simulink library "lib_energy_storage"  (Simulink 4.00)
undefined symbols (not defined in the file): air_cp, amb_tmp, cyc_mph, enable_stop, ess_cap_scale, ess_cb, ess_cc, ess_coulombic_eff, ess_init_soc, ess_max_ah_cap, ess_max_p, ess_max_p_soc, ess_max_soc, ess_max_volts, ess_min_soc, ess_min_volts, ess_MMi, ess_MMo, ess_mod_airflow, ess_mod_cp, ess_mod_cpm, ess_mod_init_tmp, ess_module_mass, ess_module_num, ess_on, ess_parallel_mod_num, ess_res_scale_coef, ess_res_scale_fun, ess_set_tmp, ess_soc, ess_th_calc, ess_th_res, ess_th_res_off, ess_th_res_on, ess_tmp, ess_voc, fund_byu, fund_byuop, mc_min_volts, saber_air_temp, Saber_Battery_IO_File, saber_init_soc, saber_init_temp, saber_init_voc, saber_k_cb, saber_k_cc, saber_k_rc, saber_k_re, saber_k_rt, saber_k_soc, t_soc, time_step
libraries: simulink3 x16, lib_energy_storage x3
(part 2 of 3)

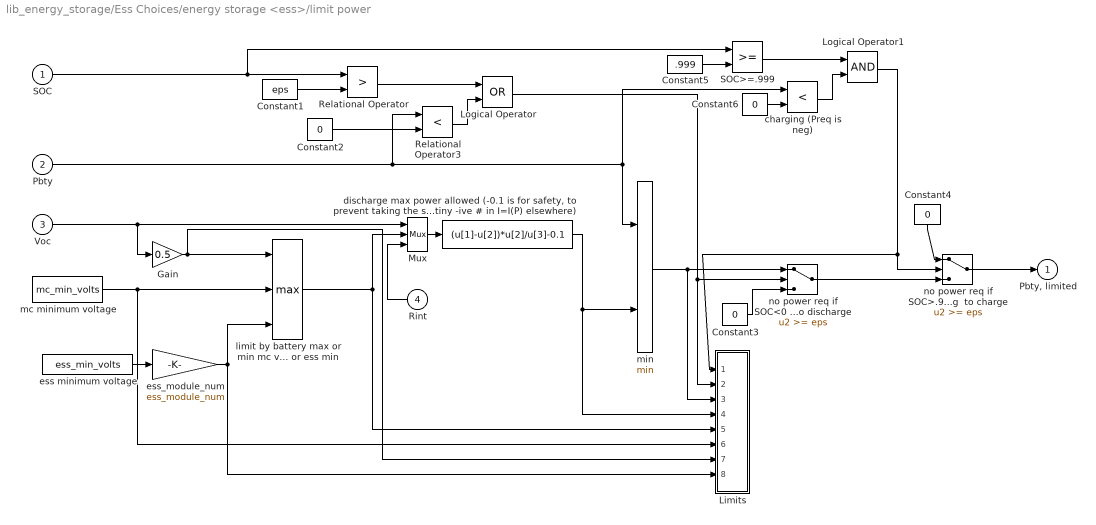
== system lib_energy_storage/Ess Choices/energy storage <ess>/limit power ==
  SOC : Inport  Port=1  LatchInput=off
  Pbty : Inport  Port=2  LatchInput=off
  Voc : Inport  Port=3  LatchInput=off
  Rint : Inport  Orientation=left  Port=4  LatchInput=off
  Constant1 : Constant  Value=eps
  Constant2 : Constant  Value=0
  Constant3 : Constant  Value=0
  Constant4 : Constant  Orientation=down  Value=0
  Constant5 : Constant  Value=.999
  Constant6 : Constant  Value=0
  Gain : Gain  Gain=0.5  Multiplication=Element-wise(K.*u)  SaturateOnIntegerOverflow=on
  Limits : Subsystem
      settings: RTWFcnNameOpts=Auto  RTWFileNameOpts=Auto
  Logical Operator : Logic  Operator=OR  Inputs=2
  Logical Operator1 : Logic  Operator=AND  Inputs=2
  Mux : Mux  Inputs=3
      settings: DisplayOption=none
  Relational Operator : RelationalOperator  Operator=>
  Relational Operator3 : RelationalOperator  Operator=<
  SOC>=.999 : RelationalOperator  Operator=>=
  charging (Preq is neg) : RelationalOperator  Operator=<
  "discharge max power allowed (-0.1 is for safety, to prevent taking the square of a tiny -ive # in I=I(P) elsewhere)" : Fcn  Expr=(u[1]-u[2])*u[2]/u[3]-0.1
  ess minimum voltage : Constant  Value=ess_min_volts
  ess_module_num : Gain  Gain=ess_module_num  Multiplication=Element-wise(K.*u)  SaturateOnIntegerOverflow=on
  limit by battery max or min mc voltage or ess min : MinMax  Function=max  Inputs=3
  mc minimum voltage : Constant  Value=mc_min_volts
  min : MinMax  Function=min  Inputs=2
  no power req if SOC<0 and trying  to discharge : Switch  Threshold=eps
  no power req if SOC>.999 and trying  to charge : Switch  Threshold=eps
  "Pbty, limited" : Outport  Port=1  InitialOutput=0
  wires:
  Logical Operator1/1 -> Limits/1(SOC  high limited), no power req if SOC>.999 and trying  to charge/2
  no power req if SOC>.999 and trying  to charge/1 -> "Pbty, limited"/1
  no power req if SOC<0 and trying  to discharge/1 -> no power req if SOC>.999 and trying  to charge/3
  Constant4/1 -> no power req if SOC>.999 and trying  to charge/1
  Constant5/1 -> SOC>=.999/2
  charging (Preq is neg)/1 -> Logical Operator1/2
  Constant6/1 -> charging (Preq is neg)/2
  SOC>=.999/1 -> Logical Operator1/1
  SOC/1 -> SOC>=.999/1, Relational Operator/1
  ess_module_num/1 -> Limits/8(V ess_min_volts), limit by battery max or min mc voltage or ess min/3
  ess minimum voltage/1 -> ess_module_num/1
  Gain/1 -> Limits/7(V battery (.5Voc)), limit by battery max or min mc voltage or ess min/1
  Rint/1 -> Mux/3
  mc minimum voltage/1 -> Limits/6(V mc_min_volts), limit by battery max or min mc voltage or ess min/2
  "discharge max power allowed (-0.1 is for safety, to prevent taking the square of a tiny -ive # in I=I(P) elsewhere)"/1 -> min/2, Limits/4(power bat limited)
  limit by battery max or min mc voltage or ess min/1 -> Limits/5(V used), Mux/2
  Mux/1 -> "discharge max power allowed (-0.1 is for safety, to prevent taking the square of a tiny -ive # in I=I(P) elsewhere)"/1
  min/1 -> Limits/3(power req), no power req if SOC<0 and trying  to discharge/1
  Voc/1 -> Gain/1, Mux/1
  Logical Operator/1 -> Limits/2(not SOC  low limited), no power req if SOC<0 and trying  to discharge/2
  Constant3/1 -> no power req if SOC<0 and trying  to discharge/3
  Relational Operator3/1 -> Logical Operator/2
  Constant2/1 -> Relational Operator3/2
  Pbty/1 -> charging (Preq is neg)/1, min/1, Relational Operator3/1
  Relational Operator/1 -> Logical Operator/1
  Constant1/1 -> Relational Operator/2

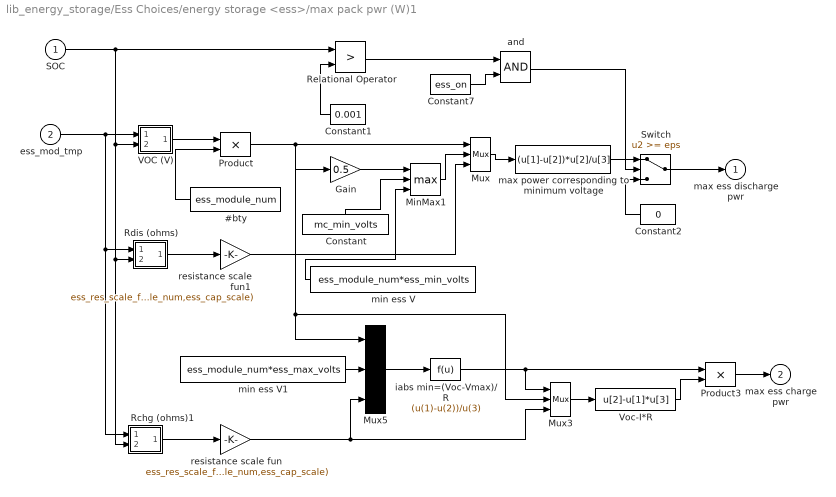
== system lib_energy_storage/Ess Choices/energy storage <ess>/max pack pwr (W)1 ==
  SOC : Inport  Port=1  LatchInput=off
  ess_mod_tmp : Inport  Port=2  LatchInput=off
  #bty : Constant  Orientation=left  Value=ess_module_num
  Constant : Constant  Orientation=up  Value=mc_min_volts
  Constant1 : Constant  Orientation=left  Value=0.001
  Constant2 : Constant  Orientation=left  Value=0
  Constant7 : Constant  Value=ess_on
  Gain : Gain  Gain=0.5  Multiplication=Element-wise(K.*u)  SaturateOnIntegerOverflow=on
  MinMax1 : MinMax  Function=max  Inputs=3
  Mux : Mux  Inputs=3
      settings: DisplayOption=none
  Mux3 : Mux  Inputs=3
      settings: DisplayOption=none
  Mux5 : Mux  Inputs=3
      settings: DisplayOption=none
  Product : Product  Inputs=2  Multiplication=Element-wise(.*)  SaturateOnIntegerOverflow=on
  Product3 : Product  Inputs=2  Multiplication=Element-wise(.*)  SaturateOnIntegerOverflow=on
  Rchg (ohms)1 : Subsystem  mask(2-D Table Lookup){@1=ess_tmp, @2=ess_soc, @3=ess_r_chg}
      mask prompts: @1 "X Index"; @2 "Y Index"; @3 "Table"
      mask help:
      | Two Dimensional Table Lookup
      | The first input corresponds to X Index and the second input corresponds to the Y Index
      mask init:
      | xindex=@1; yindex=@2; table=@3; sftab2chk(xindex,yindex,table);
      settings: RTWFcnNameOpts=Auto  RTWFileNameOpts=Auto
      mask Help: This block returns a linearly interpolated intersection from the table using the X index (which corresponds to the rows of the table) and the Y index (which corresponds to the columns of the table).  Extrapolation is used.
      mask Display: plot(-10,-10,110,110,[90,50,10],[90,40,30],[90,50,10],[50,26,20],[90,50,10],[22,13,10])
  Rdis (ohms) : Subsystem  mask(2-D Table Lookup){@1=ess_tmp, @2=ess_soc, @3=ess_r_dis}
      mask prompts: @1 "X Index"; @2 "Y Index"; @3 "Table"
      mask help:
      | Two Dimensional Table Lookup
      | The first input corresponds to X Index and the second input corresponds to the Y Index
      mask init:
      | xindex=@1; yindex=@2; table=@3; sftab2chk(xindex,yindex,table);
      settings: RTWFcnNameOpts=Auto  RTWFileNameOpts=Auto
      mask Help: This block returns a linearly interpolated intersection from the table using the X index (which corresponds to the rows of the table) and the Y index (which corresponds to the columns of the table).  Extrapolation is used.
      mask Display: plot(-10,-10,110,110,[90,50,10],[90,40,30],[90,50,10],[50,26,20],[90,50,10],[22,13,10])
  Relational Operator : RelationalOperator  Operator=>
  Switch : Switch  Threshold=eps
  VOC (V) : Subsystem  mask(2-D Table Lookup){@1=ess_tmp, @2=ess_soc, @3=ess_voc}
      mask prompts: @1 "X Index"; @2 "Y Index"; @3 "Table"
      mask help:
      | Two Dimensional Table Lookup
      | The first input corresponds to X Index and the second input corresponds to the Y Index
      mask init:
      | xindex=@1; yindex=@2; table=@3; sftab2chk(xindex,yindex,table);
      settings: RTWFcnNameOpts=Auto  RTWFileNameOpts=Auto
      mask Help: This block returns a linearly interpolated intersection from the table using the X index (which corresponds to the rows of the table) and the Y index (which corresponds to the columns of the table).  Extrapolation is used.
      mask Display: plot(-10,-10,110,110,[90,50,10],[90,40,30],[90,50,10],[50,26,20],[90,50,10],[22,13,10])
  Voc-I*R : Fcn  Expr=u[2]-u[1]*u[3]
  and : Logic  Operator=AND  Inputs=2
  iabs min=(Voc-Vmax)/R : Fcn  Expr=(u(1)-u(2))/u(3)
  max power corresponding to minimum voltage : Fcn  Expr=(u[1]-u[2])*u[2]/u[3]
  min ess V : Constant  Orientation=left  Value=ess_module_num*ess_min_volts
  min ess V1 : Constant  Value=ess_module_num*ess_max_volts
  resistance scale fun : Gain  Gain=ess_res_scale_fun(ess_res_scale_coef,ess_module_num,ess_cap_scale)  Multiplication=Element-wise(K.*u)  SaturateOnIntegerOverflow=on
  resistance scale fun1 : Gain  Gain=ess_res_scale_fun(ess_res_scale_coef,ess_module_num,ess_cap_scale)  Multiplication=Element-wise(K.*u)  SaturateOnIntegerOverflow=on
  max ess discharge pwr : Outport  Port=1  InitialOutput=0
  max ess charge pwr : Outport  Port=2  InitialOutput=0
  wires:
  Constant7/1 -> and/2
  Relational Operator/1 -> and/1
  and/1 -> Switch/2
  min ess V/1 -> MinMax1/3
  ess_mod_tmp/1 -> VOC (V)/1(x0), Rdis (ohms)/1(x0), Rchg (ohms)1/1(x0)
  Constant1/1 -> Relational Operator/2
  Constant/1 -> MinMax1/2
  Mux/1 -> max power corresponding to minimum voltage/1
  Gain/1 -> MinMax1/1
  MinMax1/1 -> Mux/2
  Product/1 -> Mux/1, Gain/1, Mux5/1, Mux3/2
  resistance scale fun1/1 -> Mux/3
  VOC (V)/1(table out) -> Product/1
  Rdis (ohms)/1(table out) -> resistance scale fun1/1
  max power corresponding to minimum voltage/1 -> Switch/1
  Constant2/1 -> Switch/3
  SOC/1 -> Relational Operator/1, VOC (V)/2(y0), Rdis (ohms)/2(y0), Rchg (ohms)1/2(y0)
  Switch/1 -> max ess discharge pwr/1
  min ess V1/1 -> Mux5/2
  Mux5/1 -> iabs min=(Voc-Vmax)/R/1
  Mux3/1 -> Voc-I*R/1
  iabs min=(Voc-Vmax)/R/1 -> Mux3/1, Product3/1
  Voc-I*R/1 -> Product3/2
  Product3/1 -> max ess charge pwr/1
  resistance scale fun/1 -> Mux5/3, Mux3/3
  Rchg (ohms)1/1(table out) -> resistance scale fun/1
  #bty/1 -> Product/2

== system lib_energy_storage/Ess Choices/energy storage <ess>/pack Voc, Rint ==
  SOC (prev) : Inport  Port=1  LatchInput=off
  req'd battery power (W) : Inport  Port=2  LatchInput=off
  mod tmp   (C) : Inport  Port=3  LatchInput=off
  #bty : Constant  Value=ess_module_num
  Product : Product  Inputs=2  Multiplication=Element-wise(.*)  SaturateOnIntegerOverflow=on
  Rchg (ohms) : Subsystem  mask(2-D Table Lookup){@1=ess_tmp, @2=ess_soc, @3=ess_r_chg}
      mask prompts: @1 "X Index"; @2 "Y Index"; @3 "Table"
      mask help:
      | Two Dimensional Table Lookup
      | The first input corresponds to X Index and the second input corresponds to the Y Index
      mask init:
      | xindex=@1; yindex=@2; table=@3; sftab2chk(xindex,yindex,table);
      settings: RTWFcnNameOpts=Auto  RTWFileNameOpts=Auto
      mask Help: This block returns a linearly interpolated intersection from the table using the X index (which corresponds to the rows of the table) and the Y index (which corresponds to the columns of the table).  Extrapolation is used.
      mask Display: plot(-10,-10,110,110,[90,50,10],[90,40,30],[90,50,10],[50,26,20],[90,50,10],[22,13,10])
  Rdis (ohms) : Subsystem  mask(2-D Table Lookup){@1=ess_tmp, @2=ess_soc, @3=ess_r_dis}
      mask prompts: @1 "X Index"; @2 "Y Index"; @3 "Table"
      mask help:
      | Two Dimensional Table Lookup
      | The first input corresponds to X Index and the second input corresponds to the Y Index
      mask init:
      | xindex=@1; yindex=@2; table=@3; sftab2chk(xindex,yindex,table);
      settings: RTWFcnNameOpts=Auto  RTWFileNameOpts=Auto
      mask Help: This block returns a linearly interpolated intersection from the table using the X index (which corresponds to the rows of the table) and the Y index (which corresponds to the columns of the table).  Extrapolation is used.
      mask Display: plot(-10,-10,110,110,[90,50,10],[90,40,30],[90,50,10],[50,26,20],[90,50,10],[22,13,10])
  Switch : Switch  Threshold=0
  VOC (V) : Subsystem  mask(2-D Table Lookup){@1=ess_tmp, @2=ess_soc, @3=ess_voc}
      mask prompts: @1 "X Index"; @2 "Y Index"; @3 "Table"
      mask help:
      | Two Dimensional Table Lookup
      | The first input corresponds to X Index and the second input corresponds to the Y Index
      mask init:
      | xindex=@1; yindex=@2; table=@3; sftab2chk(xindex,yindex,table);
      settings: RTWFcnNameOpts=Auto  RTWFileNameOpts=Auto
      mask Help: This block returns a linearly interpolated intersection from the table using the X index (which corresponds to the rows of the table) and the Y index (which corresponds to the columns of the table).  Extrapolation is used.
      mask Display: plot(-10,-10,110,110,[90,50,10],[90,40,30],[90,50,10],[50,26,20],[90,50,10],[22,13,10])
  resistance scale fun : Gain  Gain=ess_res_scale_fun(ess_res_scale_coef,ess_module_num,ess_cap_scale)  Multiplication=Element-wise(K.*u)  SaturateOnIntegerOverflow=on
  resistance scale fun1 : Gain  Gain=ess_res_scale_fun(ess_res_scale_coef,ess_module_num,ess_cap_scale)  Multiplication=Element-wise(K.*u)  SaturateOnIntegerOverflow=on
  pack open- circuit voltage : Outport  Port=1  InitialOutput=0
  pack resistance : Outport  Port=2  InitialOutput=0
  wires:
  mod tmp   (C)/1 -> Rchg (ohms)/1(x0), Rdis (ohms)/1(x0), VOC (V)/1(x0)
  SOC (prev)/1 -> Rchg (ohms)/2(y0), Rdis (ohms)/2(y0), VOC (V)/2(y0)
  req'd battery power (W)/1 -> Switch/2
  VOC (V)/1(table out) -> Product/1
  Product/1 -> pack open- circuit voltage/1
  #bty/1 -> Product/2
  Switch/1 -> pack resistance/1
  Rdis (ohms)/1(table out) -> resistance scale fun/1
  resistance scale fun/1 -> Switch/1
  Rchg (ohms)/1(table out) -> resistance scale fun1/1
  resistance scale fun1/1 -> Switch/3

== system lib_energy_storage/Ess Choices/energy storage <ess>/stop sim ==
  SOC : Inport  Port=1  LatchInput=off
  Enable : EnablePort
  Const : Constant  Orientation=up  Value=.001
  Relational Operator : RelationalOperator  Operator=<
  Stop Simulation : Stop
  wires:
  Relational Operator/1 -> Stop Simulation/1
  SOC/1 -> Relational Operator/1
  Const/1 -> Relational Operator/2

== system lib_energy_storage/Ess Choices/energy storage <ess> RC/Allow simulation to stop based on  low SOC ==
  SOC : Inport  Port=1  LatchInput=off
  Enable : EnablePort
  Const : Constant  Orientation=up  Value=.001
  Relational Operator : RelationalOperator  Operator=<
  Stop Simulation : Stop
  wires:
  Relational Operator/1 -> Stop Simulation/1
  SOC/1 -> Relational Operator/1
  Const/1 -> Relational Operator/2

== system lib_energy_storage/Ess Choices/energy storage <ess> RC/Block NOTES ==
  note: This block models the energy storage system as an SOC-dependent voltage
      | in series with an SOC- and current direction-dependent internal resistance.
      | SOC is computed assuming that A-h capacity is constant, but limited
      | such that a minimum voltage is never exceeded (replacing the
      | previous Peukert relationship which underpredicted battery capacity).
      |
      | Discharge power is limited here so as not to bring the bus (battery pack) voltage below
      | the minimum controller voltage or the minimum battery voltage and so as to allow
      | the solution of the quadratic eq'n for discharge current.
      |
      | Charge current is limited to ensure the voltage does not exceed a maximum
      | voltage
      |
      | Positive current is discharge current in the convention used here.
      | Power loss is computed as I*R+losses due to Coulombic (in)efficiency.
      |
      | Thermal modeling of the battery performance is modeled in the
      | OCV, Rint, and capacity.

== system lib_energy_storage/Ess Choices/energy storage <ess> RC/Model Parameters ==
  SOC : Inport  Port=1  LatchInput=off
  Ess Temp : Inport  Port=2  LatchInput=off
  Preq : Inport  Port=3  LatchInput=off
  Terminator : Terminator
  cb : Lookup  InputValues=ess_tmp  OutputValues=ess_cb
  cc : Lookup  InputValues=ess_tmp  OutputValues=ess_cc
  rc : Subsystem  mask(2-D Table Lookup){@1=ess_tmp, @2=ess_soc, @3=ess_rc}
      mask prompts: @1 "X Index"; @2 "Y Index"; @3 "Table"
      mask help:
      | Two Dimensional Table Lookup
      | The first input corresponds to X Index and the second input corresponds to the Y Index
      mask init:
      | xindex=@1; yindex=@2; table=@3; sftab2chk(xindex,yindex,table);
      settings: RTWFcnNameOpts=Auto  RTWFileNameOpts=Auto
      mask Help: This block returns a linearly interpolated intersection from the table using the X index (which corresponds to the rows of the table) and the Y index (which corresponds to the columns of the table).  Extrapolation is used.
      mask Display: plot(-10,-10,110,110,[90,50,10],[90,40,30],[90,50,10],[50,26,20],[90,50,10],[22,13,10])
  re : Subsystem  mask(2-D Table Lookup){@1=ess_tmp, @2=ess_soc, @3=ess_re}
      mask prompts: @1 "X Index"; @2 "Y Index"; @3 "Table"
      mask help:
      | Two Dimensional Table Lookup
      | The first input corresponds to X Index and the second input corresponds to the Y Index
      mask init:
      | xindex=@1; yindex=@2; table=@3; sftab2chk(xindex,yindex,table);
      settings: RTWFcnNameOpts=Auto  RTWFileNameOpts=Auto
      mask Help: This block returns a linearly interpolated intersection from the table using the X index (which corresponds to the rows of the table) and the Y index (which corresponds to the columns of the table).  Extrapolation is used.
      mask Display: plot(-10,-10,110,110,[90,50,10],[90,40,30],[90,50,10],[50,26,20],[90,50,10],[22,13,10])
  rt : Subsystem  mask(2-D Table Lookup){@1=ess_tmp, @2=ess_soc, @3=ess_rt}
      mask prompts: @1 "X Index"; @2 "Y Index"; @3 "Table"
      mask help:
      | Two Dimensional Table Lookup
      | The first input corresponds to X Index and the second input corresponds to the Y Index
      mask init:
      | xindex=@1; yindex=@2; table=@3; sftab2chk(xindex,yindex,table);
      settings: RTWFcnNameOpts=Auto  RTWFileNameOpts=Auto
      mask Help: This block returns a linearly interpolated intersection from the table using the X index (which corresponds to the rows of the table) and the Y index (which corresponds to the columns of the table).  Extrapolation is used.
      mask Display: plot(-10,-10,110,110,[90,50,10],[90,40,30],[90,50,10],[50,26,20],[90,50,10],[22,13,10])
  Cb : Outport  Port=1  InitialOutput=0
  Cc : Outport  Port=2  InitialOutput=0
  Re : Outport  Port=3  InitialOutput=0
  Rc : Outport  Port=4  InitialOutput=0
  Rt : Outport  Port=5  InitialOutput=0
  wires:
  rc/1(table out) -> Rc/1
  rt/1(table out) -> Rt/1
  re/1(table out) -> Re/1
  cc/1 -> Cc/1
  cb/1 -> Cb/1
  SOC/1 -> rt/2(y0), rc/2(y0), re/2(y0)
  Preq/1 -> Terminator/1
  Ess Temp/1 -> rt/1(x0), rc/1(x0), re/1(x0), cc/1, cb/1

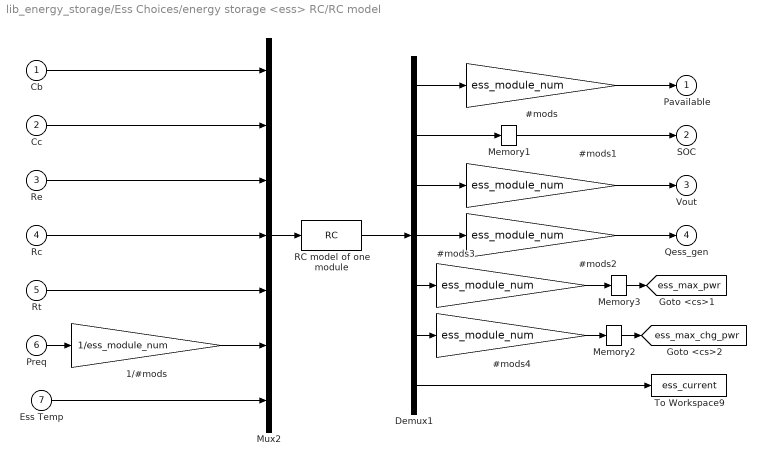
== system lib_energy_storage/Ess Choices/energy storage <ess> RC/RC model ==
  Cb : Inport  Port=1  LatchInput=off
  Cc : Inport  Port=2  LatchInput=off
  Re : Inport  Port=3  LatchInput=off
  Rc : Inport  Port=4  LatchInput=off
  Rt : Inport  Port=5  LatchInput=off
  Preq : Inport  Port=6  LatchInput=off
  Ess Temp : Inport  Port=7  LatchInput=off
  #mods{,1..4} (5 alike) : Gain  Gain=ess_module_num  Multiplication=Element-wise(K.*u)  SaturateOnIntegerOverflow=on
  1/#mods : Gain  Gain=1/ess_module_num  Multiplication=Element-wise(K.*u)  SaturateOnIntegerOverflow=on
  Demux1 : Demux  Outputs=7  BusSelectionMode=off
  Memory1 : Memory  X0=ess_init_soc  InheritSampleTime=off
      settings: RTWStateStorageClass=Auto
  Memory2 : Memory  X0=0  InheritSampleTime=off
      settings: RTWStateStorageClass=Auto
  Memory3 : Memory  X0=0  InheritSampleTime=off
      settings: RTWStateStorageClass=Auto
  Mux2 : Mux  Inputs=7
      settings: DisplayOption=none
  RC model of one module : S-Function  FunctionName=RC  Parameters=ess_min_volts,ess_max_volts,mc_min_volts/ess_module_num,ess_soc,ess_tmp,ess_voc,ess_init_soc,ess_mod_init_tmp  PortCounts=[]  SFunctionModules=''
  To Workspace9 : ToWorkspace  VariableName=ess_current  SampleTime=-1  SaveFormat=Array
  Pavailable : Outport  Port=1  InitialOutput=0
  SOC : Outport  Port=2  InitialOutput=0
  Vout : Outport  Port=3  InitialOutput=0
  Qess_gen : Outport  Port=4  InitialOutput=0
  tag scope: ess_max_chg_pwr=global, ess_max_pwr=global
  wires:
  RC model of one module/1 -> Demux1/1
  #mods2/1 -> Qess_gen/1
  Demux1/4 -> #mods2/1
  #mods1/1 -> Vout/1
  Demux1/3 -> #mods1/1
  #mods/1 -> Pavailable/1
  Demux1/1 -> #mods/1
  1/#mods/1 -> Mux2/6
  Preq/1 -> 1/#mods/1
  Mux2/1 -> RC model of one module/1
  Rt/1 -> Mux2/5
  Rc/1 -> Mux2/4
  Re/1 -> Mux2/3
  Cc/1 -> Mux2/2
  Cb/1 -> Mux2/1
  Ess Temp/1 -> Mux2/7
  Demux1/7 -> To Workspace9/1
  Demux1/6 -> #mods4/1
  Memory2/1 -> [ess_max_chg_pwr]
  Demux1/5 -> #mods3/1
  Memory3/1 -> [ess_max_pwr]
  Demux1/2 -> Memory1/1
  Memory1/1 -> SOC/1
  #mods3/1 -> Memory3/1
  #mods4/1 -> Memory2/1

== system lib_energy_storage/Ess Choices/energy storage <ess> RC/Thermal Model of Battery ==
  Qess_gen : Inport  Port=1  LatchInput=off
  Enable : EnablePort  StatesWhenEnabling=reset
  #of mods : Gain  Gain=ess_module_num  Multiplication=Element-wise(K.*u)  SaturateOnIntegerOverflow=on
  1/#of mods : Gain  Gain=1/ess_module_num  Multiplication=Element-wise(K.*u)  SaturateOnIntegerOverflow=on
  1/mcp : Gain  Gain=1/(ess_module_mass*ess_mod_cp)  Multiplication=Element-wise(K.*u)  SaturateOnIntegerOverflow=on
  Block NOTES : Subsystem
      settings: RTWFcnNameOpts=Auto  RTWFileNameOpts=Auto
      mask Display: disp('Block\nNOTES')
  Memory : Memory  Orientation=left  X0=cyc_mph(1,2)*.447  InheritSampleTime=off
      settings: RTWStateStorageClass=Auto
  Memory1 : Memory  Orientation=left  X0=cyc_mph(1,2)*.447  InheritSampleTime=off
      settings: RTWStateStorageClass=Auto
  Mux20 : Mux  Inputs=3
      settings: DisplayOption=none
  Qc : Sum  Inputs=++  SaturateOnIntegerOverflow=on
  Qess_case : Fcn  Expr=(u(2) - u(1))/u(3)
  Saturation3 : Saturate  Orientation=left  UpperLimit=1  LowerLimit=0  LinearizeAsGain=on
  Tair,ave : Subsystem  TreatAsAtomicUnit=on
      settings: RTWFcnNameOpts=Auto  RTWFileNameOpts=Auto
  Tess2 : Integrator  ExternalReset=none  InitialConditionSource=internal  InitialCondition=ess_mod_init_tmp  LimitOutput=off  UpperSaturationLimit=inf  LowerSaturationLimit=-inf  ShowSaturationPort=off  ShowStatePort=off  AbsoluteTolerance=auto
  thermostat : Fcn  Orientation=left  Expr=u(1) - ess_set_tmp
  Tess : Outport  Port=1  InitialOutput=0
  Tair : Outport  Port=2
  Qair : Outport  Port=3  OutputWhenDisabled=reset  InitialOutput=0
  wires:
  Tair,ave/1(Tair_ave) -> Tair/1, Mux20/2
  Tair,ave/2(Th Res) -> Mux20/3
  Mux20/1 -> Qess_case/1
  #of mods/1 -> Qair/1
  Memory/1 -> Tair,ave/1(Qess_case)
  Memory1/1 -> Tair,ave/Enable
  Saturation3/1 -> Memory1/1
  thermostat/1 -> Saturation3/1
  1/#of mods/1 -> Qc/2
  Qess_gen/1 -> 1/#of mods/1
  Tess2/1 -> thermostat/1, Mux20/1, Tess/1
  1/mcp/1 -> Tess2/1
  Qess_case/1 -> #of mods/1, Memory/1, Qc/1
  Qc/1 -> 1/mcp/1

== system lib_energy_storage/Ess Choices/energy storage <ess> RC/documentation9 ==

== system lib_energy_storage/Ess Choices/energy storage <ess> nnet/Limits ==
  power req : Inport  Port=1  LatchInput=off
  power  available from battery : Inport  Port=2  LatchInput=off
  Const{1..4} (4 alike) : Constant  Value=0
  Relational Operator1 : RelationalOperator  Operator===
  limited by battery : Logic  Operator=NOT  Inputs=1
  tag scope: ess_maxV_limited=global, ess_minV_limited=global, ess_pwr_limited=global, ess_soc_limited=global, mc_voltage_limited=global
  wires:
  Relational Operator1/1 -> limited by battery/1
  limited by battery/1 -> [ess_pwr_limited]
  power req/1 -> Relational Operator1/1
  power  available from battery/1 -> Relational Operator1/2
  Const4/1 -> [mc_voltage_limited]
  Const3/1 -> [ess_minV_limited]
  Const2/1 -> [ess_maxV_limited]
  Const1/1 -> [ess_soc_limited]

== system lib_energy_storage/Ess Choices/energy storage <ess> nnet/NNet ==
  Preq : Inport  Port=1  LatchInput=off
  SOC : Inport  Port=2  LatchInput=off
  Enable : EnablePort
  De-Normalizer1 Voltage : Fcn  Expr=(u-0.2)*(ess_MMo(2,2)-ess_MMo(2,1))/(0.8-0.2)+ess_MMo(2,1)
  De-Normalizer2 Current : Fcn  Expr=(u-0.2)*(ess_MMo(1,2)-ess_MMo(1,1))/(0.8-0.2)+ess_MMo(1,1)
  Demux : Demux  Outputs=2  BusSelectionMode=off
  Mux : Mux  Inputs=2
      settings: DisplayOption=none
  Neural Network : Subsystem
      settings: RTWFcnNameOpts=Auto  RTWFileNameOpts=Auto
  Normalizer Power : Fcn  Expr=(u-ess_MMi(1,1))/(ess_MMi(1,2)-ess_MMi(1,1))
  Normalizer SOC : Fcn  Expr=(u-ess_MMi(2,1))/(ess_MMi(2,2)-ess_MMi(2,1))
  V : Outport  Port=1  InitialOutput=0
  i : Outport  Port=2  OutputWhenDisabled=reset  InitialOutput=0
  wires:
  De-Normalizer1 Voltage/1 -> V/1
  Demux/2 -> De-Normalizer1 Voltage/1
  Demux/1 -> De-Normalizer2 Current/1
  De-Normalizer2 Current/1 -> i/1
  Normalizer SOC/1 -> Mux/2
  SOC/1 -> Normalizer SOC/1
  Normalizer Power/1 -> Mux/1
  Preq/1 -> Normalizer Power/1
  Neural Network/1("y{1}") -> Demux/1
  Mux/1 -> Neural Network/1("p{1}")

== system lib_energy_storage/Ess Choices/energy storage <ess> nnet/No Thermal model ==
  Const1 : Constant  Value=0
  Const2 : Constant  Value=amb_tmp
  Const3 : Constant  Value=0
  To WS1 : ToWorkspace  VariableName=ess_pwr_loss_a  SampleTime=0  SaveFormat=Array
  To WS2 : ToWorkspace  VariableName=ess_mod_tmp  SampleTime=0  SaveFormat=Array
  To WS3 : ToWorkspace  VariableName=ess_air_tmp  SampleTime=0  SaveFormat=Array
  To WS4 : ToWorkspace  VariableName=ess_air_th_pwr  SampleTime=0  SaveFormat=Array
  wires:
  Const3/1 -> To WS4/1
  Const2/1 -> To WS3/1, To WS2/1
  Const1/1 -> To WS1/1

== system lib_energy_storage/Ess Choices/energy storage <ess> nnet/SOC algorithm ==
  note: SOC=(Max Ah capacity-Ah used)/Max Ah capacity
  (A) : Inport  Port=1  LatchInput=off
  tmp (C) : Inport  Port=2  LatchInput=off
  (sec->hrs) : Gain  Gain=1/3600  Multiplication=Element-wise(K.*u)  SaturateOnIntegerOverflow=on
  0 <= SOC <= 1 : Saturate  UpperLimit=1  LowerLimit=0  LinearizeAsGain=on
  A-h remaining : Sum  Inputs=-+  SaturateOnIntegerOverflow=on
  Ah used : Integrator  ExternalReset=none  InitialConditionSource=external  InitialCondition=(1-ess_init_soc)*ess_max_ah_cap  LimitOutput=off  UpperSaturationLimit=inf  LowerSaturationLimit=-inf  ShowSaturationPort=off  ShowStatePort=off  AbsoluteTolerance=auto
  Fcn : Fcn  Expr=1/u
  Fcn1 : Fcn  Expr=(1-ess_init_soc)*u
  SOC : Product  Inputs=2  Multiplication=Element-wise(.*)  SaturateOnIntegerOverflow=on
  Switch : Switch  Threshold=0
  adjusted A : Product  Inputs=2  Multiplication=Element-wise(.*)  SaturateOnIntegerOverflow=on
  coul eff : Lookup  InputValues=ess_tmp  OutputValues=ess_coulombic_eff
  max cap : Lookup  InputValues=ess_tmp  OutputValues=ess_max_ah_cap
  SOC1 : Outport  Port=1  InitialOutput=0
  wires:
  Fcn1/1 -> Ah used/2
  max cap/1 -> Fcn1/1, Fcn/1, A-h remaining/2
  adjusted A/1 -> Switch/3
  coul eff/1 -> adjusted A/2
  tmp (C)/1 -> coul eff/1, max cap/1
  0 <= SOC <= 1/1 -> SOC1/1
  A-h remaining/1 -> SOC/1
  SOC/1 -> 0 <= SOC <= 1/1
  Fcn/1 -> SOC/2
  Ah used/1 -> A-h remaining/1
  (sec->hrs)/1 -> Ah used/1
  Switch/1 -> (sec->hrs)/1
  (A)/1 -> adjusted A/1, Switch/1, Switch/2

== system lib_energy_storage/Ess Choices/energy storage <ess> nnet/max pack pwr (W) ==
  SOC : Inport  Port=1  LatchInput=off
  # batteries : Gain  Gain=ess_module_num  Multiplication=Element-wise(K.*u)  SaturateOnIntegerOverflow=on
  max power : Lookup  InputValues=ess_max_p_soc  OutputValues=ess_max_p
  ess discharge pwr : Outport  Port=1  InitialOutput=0
  wires:
  # batteries/1 -> ess discharge pwr/1
  max power/1 -> # batteries/1
  SOC/1 -> max power/1

== system lib_energy_storage/Ess Choices/energy storage <ess> nnet/stop sim ==
  SOC : Inport  Port=1  LatchInput=off
  Enable : EnablePort
  Const : Constant  Orientation=up  Value=.001
  Relational Operator : RelationalOperator  Operator=<
  Stop Simulation : Stop
  wires:
  Relational Operator/1 -> Stop Simulation/1
  SOC/1 -> Relational Operator/1
  Const/1 -> Relational Operator/2

== system lib_energy_storage/Ess Choices/energy storage <ess> Saber/Block NOTES ==
  note: Saber co-simulation

== system lib_energy_storage/Ess Choices/energy storage <ess> Saber/Power ==
  Current : Inport  Port=1  LatchInput=off
  Voltage : Inport  Port=2  LatchInput=off
  P=i*V : Product  Inputs=2  Multiplication=Element-wise(.*)  SaturateOnIntegerOverflow=on
  To Workspace9 : ToWorkspace  VariableName=ess_pwr_out_a  SampleTime=-1  SaveFormat=Array
  Avail Power : Outport  Port=1
  wires:
  P=i*V/1 -> Avail Power/1, To Workspace9/1
  Current/1 -> P=i*V/1
  Voltage/1 -> P=i*V/2

== system lib_energy_storage/Ess Choices/energy storage <ess> Saber/Power request ==
  power req'd : Inport  Port=1  LatchInput=off
  1/# batteries : Gain  Gain=1/ess_module_num  Multiplication=Element-wise(K.*u)  SaturateOnIntegerOverflow=on
  Relational Operator1 : RelationalOperator  Operator===
  To Workspace8 : ToWorkspace  VariableName=ess_pwr_out_r  SampleTime=-1  SaveFormat=Array
  if P==0 : Constant  Value=0
  "if P==0, pass  P=0.0001" : Switch  Threshold=0.1
  non-zero power : Constant  Value=0.0001
  P request : Outport  Port=1
  wires:
  power req'd/1 -> To Workspace8/1, 1/# batteries/1
  1/# batteries/1 -> "if P==0, pass  P=0.0001"/3, Relational Operator1/2
  "if P==0, pass  P=0.0001"/1 -> P request/1
  if P==0/1 -> Relational Operator1/1
  non-zero power/1 -> "if P==0, pass  P=0.0001"/1
  Relational Operator1/1 -> "if P==0, pass  P=0.0001"/2

== system lib_energy_storage/Ess Choices/energy storage <ess> Saber/SOC's ==
  Saber SOC's : Inport  Orientation=down  Port=1  LatchInput=off
  Const : Constant  Orientation=down  Value=enable_stop
  Mean : Subsystem
      settings: RTWFcnNameOpts=Auto  RTWFileNameOpts=Auto
  To Workspace2 : ToWorkspace  VariableName=saber_ess_SOC  SampleTime=-1  SaveFormat=Array
  soc mem : Memory  X0=ess_init_soc  InheritSampleTime=off
      settings: RTWStateStorageClass=Auto
  stop sim : Subsystem  TreatAsAtomicUnit=on
      settings: RTWFcnNameOpts=Auto  RTWFileNameOpts=Auto
  tag scope: SOC=global
  wires:
  Saber SOC's/1 -> Mean/1(In), To Workspace2/1
  Const/1 -> stop sim/Enable
  Mean/1(Out) -> soc mem/1
  soc mem/1 -> [SOC], stop sim/1(SOC)

== system lib_energy_storage/Ess Choices/energy storage <ess> Saber/Temps ==
  Saber Temps : Inport  Orientation=down  Port=1  LatchInput=off
  Mean : Subsystem
      settings: RTWFcnNameOpts=Auto  RTWFileNameOpts=Auto
  To WS2 : ToWorkspace  VariableName=ess_mod_tmp  SampleTime=0  SaveFormat=Array
  To Workspace3 : ToWorkspace  VariableName=saber_ess_temp  SampleTime=-1  SaveFormat=Array
  wires:
  Saber Temps/1 -> Mean/1(In), To Workspace3/1
  Mean/1(Out) -> To WS2/1

== system lib_energy_storage/Ess Choices/energy storage <ess> Saber/Thermal Power ==
  Saber Thermal P : Inport  Port=1  LatchInput=off
  # batteries : Gain  Gain=ess_module_num  Multiplication=Element-wise(K.*u)  SaturateOnIntegerOverflow=on
  Saturation : Saturate  UpperLimit=inf  LowerLimit=0  LinearizeAsGain=on
  Sum2 : Sum  Inputs=1  SaturateOnIntegerOverflow=on
  To Workspace3 : ToWorkspace  VariableName=saber_ess_th_pwr  SampleTime=-1  SaveFormat=Array
  To Workspace9 : ToWorkspace  VariableName=ess_pwr_loss_a  SampleTime=-1  SaveFormat=Array
  wires:
  Sum2/1 -> To Workspace9/1
  # batteries/1 -> Sum2/1, To Workspace3/1
  Saber Thermal P/1 -> Saturation/1
  Saturation/1 -> # batteries/1

== system lib_energy_storage/Ess Choices/energy storage <ess> Saber/Time Dependent Power Request ==
  P request : Inport  Port=1  LatchInput=off
  Constant : Constant  Value=0
  Enabled Subsystem1 : Subsystem  TreatAsAtomicUnit=on
      settings: RTWFcnNameOpts=Auto  RTWFileNameOpts=Auto
  IC : InitialCondition  Value=time_step
  Matrix Concatenation1 : lib_energy_storage/Ess Choices/energy storage <ess> Saber/Matrix Concatenation1  numInports=6  catMethod=Horizontal
  Memory1 : Memory  X0=.001  InheritSampleTime=on
      settings: RTWStateStorageClass=Auto
  Memory2 : Memory  X0=80  InheritSampleTime=on
      settings: RTWStateStorageClass=Auto
  Relational Operator : RelationalOperator  Operator===
  Saturation : Saturate  UpperLimit=inf  LowerLimit=.001  LinearizeAsGain=on
  P request time : Outport  Port=1
  wires:
  Relational Operator/1 -> Enabled Subsystem1/Enable
  [time] -> Relational Operator/2
  Enabled Subsystem1/1(Out1) -> Matrix Concatenation1/2
  Memory2/1 -> Matrix Concatenation1/4
  Matrix Concatenation1/1 -> P request time/1
  IC/1 -> Matrix Concatenation1/5
  Saturation/1 -> Memory1/1
  [time] -> Saturation/1
  Memory1/1 -> Matrix Concatenation1/3
  [time] -> IC/1
  Constant/1 -> Relational Operator/1, Matrix Concatenation1/1
  P request/1 -> Memory2/1, Matrix Concatenation1/6, Enabled Subsystem1/1(In1)  "P request"

== system lib_energy_storage/Ess Choices/energy storage <ess> Saber/Voltages ==
  Saber Voltages : Inport  Port=1  LatchInput=off
  # batteries : Gain  Gain=ess_module_num  Multiplication=Element-wise(K.*u)  SaturateOnIntegerOverflow=on
  Sum : Sum  Inputs=1  SaturateOnIntegerOverflow=on
  To Workspace1 : ToWorkspace  VariableName=ess_voltage  SampleTime=-1  SaveFormat=Array
  To Workspace11 : ToWorkspace  VariableName=saber_ess_voltage  SampleTime=-1  SaveFormat=Array
  ADV Voltage : Outport  Port=1
  tag scope: bus_voltage=global
  wires:
  # batteries/1 -> Sum/1, To Workspace11/1
  Sum/1 -> [bus_voltage], To Workspace1/1, ADV Voltage/1
  Saber Voltages/1 -> # batteries/1

== system lib_energy_storage/Ess Choices/energy storage <ess> Saber/max pack pwr (W) ==
  note: Edit in the future
      | Used in series power follower
  Ground : Ground
  tag scope: ess_max_pwr=global
  wires:
  Ground/1 -> [ess_max_pwr]

== system lib_energy_storage/Ess Choices/energy storage <ess> fundamental model/Block NOTES ==
  note: Fundamentally based SOC model developed at BYU
      | Files needed:
      | input1.dat
      | input2.dat
      | input3.dat
      | nrel13cs.dll

== system lib_energy_storage/Ess Choices/energy storage <ess> fundamental model/ess tmp ==
  Qess_gen : Inport  Port=1  LatchInput=off
  Enable : EnablePort  StatesWhenEnabling=reset
  #of mods : Gain  Gain=ess_module_num  Multiplication=Element-wise(K.*u)  SaturateOnIntegerOverflow=on
  1/#of mods : Gain  Gain=1/ess_module_num  Multiplication=Element-wise(K.*u)  SaturateOnIntegerOverflow=on
  1/mcp : Gain  Gain=1/(ess_module_mass*ess_mod_cp)  Multiplication=Element-wise(K.*u)  SaturateOnIntegerOverflow=on
  Block NOTES : Subsystem
      settings: RTWFcnNameOpts=Auto  RTWFileNameOpts=Auto
      mask Display: disp('Block\nNOTES')
  Memory : Memory  Orientation=left  X0=cyc_mph(1,2)*.447  InheritSampleTime=off
      settings: RTWStateStorageClass=Auto
  Memory1 : Memory  Orientation=left  X0=cyc_mph(1,2)*.447  InheritSampleTime=off
      settings: RTWStateStorageClass=Auto
  Mux20 : Mux  Inputs=3
      settings: DisplayOption=none
  Qc : Sum  Inputs=++  SaturateOnIntegerOverflow=on
  Qess_case : Fcn  Expr=(u(2) - u(1))/u(3)
  Saturation3 : Saturate  Orientation=left  UpperLimit=1  LowerLimit=0  LinearizeAsGain=on
  Tair,ave : Subsystem  TreatAsAtomicUnit=on
      settings: RTWFcnNameOpts=Auto  RTWFileNameOpts=Auto
  Tess2 : Integrator  ExternalReset=none  InitialConditionSource=internal  InitialCondition=ess_mod_init_tmp  LimitOutput=off  UpperSaturationLimit=inf  LowerSaturationLimit=-inf  ShowSaturationPort=off  ShowStatePort=off  AbsoluteTolerance=auto
  thermostat : Fcn  Orientation=left  Expr=u(1) - ess_set_tmp
  Tess : Outport  Port=1  InitialOutput=0
  Tair : Outport  Port=2
  Qair : Outport  Port=3  OutputWhenDisabled=reset  InitialOutput=0
  wires:
  Tair,ave/1(Tair_ave) -> Tair/1, Mux20/2
  Tair,ave/2(Th Res) -> Mux20/3
  Mux20/1 -> Qess_case/1
  #of mods/1 -> Qair/1
  Memory/1 -> Tair,ave/1(Qess_case)
  Memory1/1 -> Tair,ave/Enable
  Saturation3/1 -> Memory1/1
  thermostat/1 -> Saturation3/1
  1/#of mods/1 -> Qc/2
  Qess_gen/1 -> 1/#of mods/1
  Tess2/1 -> thermostat/1, Mux20/1, Tess/1
  1/mcp/1 -> Tess2/1
  Qess_case/1 -> #of mods/1, Memory/1, Qc/1
  Qc/1 -> 1/mcp/1

== system lib_energy_storage/Ess Choices/energy storage <ess> fundamental model/max pack pwr (W) ==
  SOC : Inport  Port=1  LatchInput=off
  # batteries : Gain  Gain=ess_module_num  Multiplication=Element-wise(K.*u)  SaturateOnIntegerOverflow=on
  max power : Lookup  InputValues=ess_max_p_soc  OutputValues=ess_max_p
  ess discharge pwr : Outport  Port=1  InitialOutput=0
  wires:
  # batteries/1 -> ess discharge pwr/1
  max power/1 -> # batteries/1
  SOC/1 -> max power/1

== system lib_energy_storage/Ess Choices/energy storage <ess> fundamental model/stop sim ==
  SOC : Inport  Port=1  LatchInput=off
  Enable : EnablePort
  Const : Constant  Orientation=up  Value=0.1
  Relational Operator : RelationalOperator  Operator=<
  Stop Simulation : Stop
  wires:
  Relational Operator/1 -> Stop Simulation/1
  SOC/1 -> Relational Operator/1
  Const/1 -> Relational Operator/2

== system lib_energy_storage/Ess Choices/energy storage <ess> optima fundamental model/Block NOTES ==
  note: Fundamentally based SOC model developed at BYU
      | Files needed:
      | input1.dat
      | input2.dat
      | input3.dat
      | nrel13cs.dll

== system lib_energy_storage/Ess Choices/energy storage <ess> optima fundamental model/ess tmp ==
  Qess_gen : Inport  Port=1  LatchInput=off
  Enable : EnablePort  StatesWhenEnabling=reset
  #of mods : Gain  Gain=ess_module_num  Multiplication=Element-wise(K.*u)  SaturateOnIntegerOverflow=on
  1/#of mods : Gain  Gain=1/ess_module_num  Multiplication=Element-wise(K.*u)  SaturateOnIntegerOverflow=on
  1/mcp : Gain  Gain=1/(ess_module_mass*ess_mod_cp)  Multiplication=Element-wise(K.*u)  SaturateOnIntegerOverflow=on
  Block NOTES : Subsystem
      settings: RTWFcnNameOpts=Auto  RTWFileNameOpts=Auto
      mask Display: disp('Block\nNOTES')
  Memory : Memory  Orientation=left  X0=cyc_mph(1,2)*.447  InheritSampleTime=off
      settings: RTWStateStorageClass=Auto
  Memory1 : Memory  Orientation=left  X0=cyc_mph(1,2)*.447  InheritSampleTime=off
      settings: RTWStateStorageClass=Auto
  Mux20 : Mux  Inputs=3
      settings: DisplayOption=none
  Qc : Sum  Inputs=++  SaturateOnIntegerOverflow=on
  Qess_case : Fcn  Expr=(u(2) - u(1))/u(3)
  Saturation3 : Saturate  Orientation=left  UpperLimit=1  LowerLimit=0  LinearizeAsGain=on
  Tair,ave : Subsystem  TreatAsAtomicUnit=on
      settings: RTWFcnNameOpts=Auto  RTWFileNameOpts=Auto
  Tess2 : Integrator  ExternalReset=none  InitialConditionSource=internal  InitialCondition=ess_mod_init_tmp  LimitOutput=off  UpperSaturationLimit=inf  LowerSaturationLimit=-inf  ShowSaturationPort=off  ShowStatePort=off  AbsoluteTolerance=auto
  thermostat : Fcn  Orientation=left  Expr=u(1) - ess_set_tmp
  Tess : Outport  Port=1  InitialOutput=0
  Tair : Outport  Port=2
  Qair : Outport  Port=3  OutputWhenDisabled=reset  InitialOutput=0
  wires:
  Tair,ave/1(Tair_ave) -> Tair/1, Mux20/2
  Tair,ave/2(Th Res) -> Mux20/3
  Mux20/1 -> Qess_case/1
  #of mods/1 -> Qair/1
  Memory/1 -> Tair,ave/1(Qess_case)
  Memory1/1 -> Tair,ave/Enable
  Saturation3/1 -> Memory1/1
  thermostat/1 -> Saturation3/1
  1/#of mods/1 -> Qc/2
  Qess_gen/1 -> 1/#of mods/1
  Tess2/1 -> thermostat/1, Mux20/1, Tess/1
  1/mcp/1 -> Tess2/1
  Qess_case/1 -> #of mods/1, Memory/1, Qc/1
  Qc/1 -> 1/mcp/1

== system lib_energy_storage/Ess Choices/energy storage <ess> optima fundamental model/max pack pwr (W) ==
  SOC : Inport  Port=1  LatchInput=off
  # batteries : Gain  Gain=ess_module_num  Multiplication=Element-wise(K.*u)  SaturateOnIntegerOverflow=on
  max power : Lookup  InputValues=ess_max_p_soc  OutputValues=ess_max_p
  ess discharge pwr : Outport  Port=1  InitialOutput=0
  wires:
  # batteries/1 -> ess discharge pwr/1
  max power/1 -> # batteries/1
  SOC/1 -> max power/1

== system lib_energy_storage/Ess Choices/energy storage <ess> optima fundamental model/stop sim ==
  SOC : Inport  Port=1  LatchInput=off
  Enable : EnablePort
  Const : Constant  Orientation=up  Value=.001
  Relational Operator : RelationalOperator  Operator=<
  Stop Simulation : Stop
  wires:
  Relational Operator/1 -> Stop Simulation/1
  SOC/1 -> Relational Operator/1
  Const/1 -> Relational Operator/2

== system lib_energy_storage/Ess Choices/Ultracapacitor  System/Calc Iout/SOC limit ==
  SOC : Inport  Port=1  LatchInput=off
  Pbty : Inport  Port=2  LatchInput=off
  Constant1 : Constant  Value=0.001
  Constant5 : Constant  Value=.999
  Constant9 : Constant  Value=0
  Logical Operator : Logic  Operator=OR  Inputs=2
  Logical Operator1 : Logic  Operator=AND  Inputs=2
  Logical Operator2 : Logic  Operator=NOT  Inputs=1
  Relational Operator : RelationalOperator  Operator=>
  Relational Operator3 : RelationalOperator  Operator=<
  SOC>=.999 : RelationalOperator  Operator=>=
  charging (Preq is neg) : RelationalOperator  Operator=<
  no power req if SOC<0 and trying  to discharge : Switch  Threshold=eps
  no power req if SOC>.999 and trying  to charge : Switch  Threshold=eps
  "Pbty, limited" : Outport  Port=1  InitialOutput=0
  tag scope: ess_soc_hi_limited=global, ess_soc_low_limited=global
  wires:
  Constant1/1 -> Relational Operator/2
  Pbty/1 -> Relational Operator3/1, charging (Preq is neg)/1, no power req if SOC<0 and trying  to discharge/1
  Logical Operator/1 -> Logical Operator2/1, no power req if SOC<0 and trying  to discharge/2
  SOC/1 -> Relational Operator/1, SOC>=.999/1
  SOC>=.999/1 -> Logical Operator1/1
  charging (Preq is neg)/1 -> Logical Operator1/2
  Constant5/1 -> SOC>=.999/2
  no power req if SOC<0 and trying  to discharge/1 -> no power req if SOC>.999 and trying  to charge/3
  no power req if SOC>.999 and trying  to charge/1 -> "Pbty, limited"/1
  Logical Operator1/1 -> [ess_soc_hi_limited], no power req if SOC>.999 and trying  to charge/2
  Relational Operator3/1 -> Logical Operator/2
  Constant9/1 -> Relational Operator3/2, charging (Preq is neg)/2, no power req if SOC<0 and trying  to discharge/3, no power req if SOC>.999 and trying  to charge/1
  Relational Operator/1 -> Logical Operator/1
  Logical Operator2/1 -> [ess_soc_low_limited]

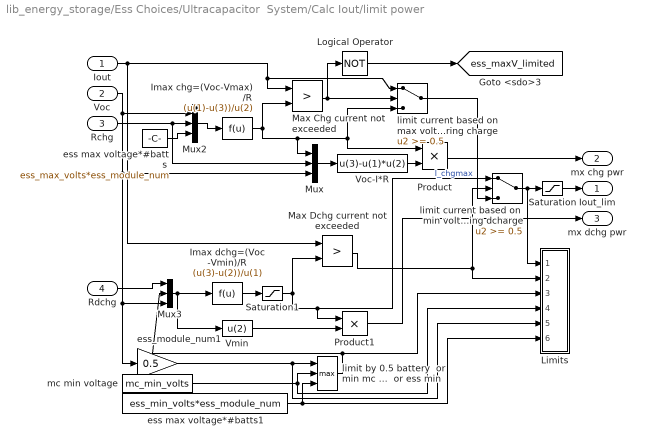
== system lib_energy_storage/Ess Choices/Ultracapacitor  System/Calc Iout/limit power ==
  Iout : Inport  Port=1  LatchInput=off
  Voc : Inport  Port=2  LatchInput=off
  Rchg : Inport  Port=3  LatchInput=off
  Rdchg : Inport  Port=4  LatchInput=off
  Imax chg=(Voc-Vmax)/R : Fcn  Expr=(u(1)-u(3))/u(2)
  Imax dchg=(Voc -Vmin)/R : Fcn  Expr=(u(3)-u(2))/u(1)
  Limits : Subsystem
      settings: RTWFcnNameOpts=Auto  RTWFileNameOpts=Auto
  Logical Operator : Logic  Operator=NOT  Inputs=2
  Max Chg current not exceeded : RelationalOperator  Operator=>
  Max Dchg current not exceeded : RelationalOperator  Operator=>
  Mux : Mux  Inputs=3
  Mux2 : Mux  Inputs=3
  Mux3 : Mux  Inputs=3
  Product : Product  Inputs=2  Multiplication=Element-wise(.*)  SaturateOnIntegerOverflow=on
  Product1 : Product  Inputs=2  Multiplication=Element-wise(.*)  SaturateOnIntegerOverflow=on
  Saturation : Saturate  UpperLimit=625*ess_parallel_mod_num  LowerLimit=-625*ess_parallel_mod_num  LinearizeAsGain=on
  Saturation1 : Saturate  UpperLimit=inf  LowerLimit=0  LinearizeAsGain=on
  Vmin : Fcn  Expr=u(2)
  Voc-I*R : Fcn  Expr=u(3)-u(1)*u(2)
  ess max voltage*#batts : Constant  Value=ess_max_volts*ess_module_num
  ess max voltage*#batts1 : Constant  Value=ess_min_volts*ess_module_num
  ess_module_num1 : Gain  Gain=0.5  Multiplication=Element-wise(K.*u)  SaturateOnIntegerOverflow=on
  limit by 0.5 battery  or min mc voltage  or ess min : MinMax  Function=max  Inputs=3
  limit current based on  max voltage during charge : Switch  Threshold=0.5
  limit current based on  min voltage during dcharge : Switch  Threshold=0.5
  mc min voltage : Constant  Value=mc_min_volts
  Iout_lim : Outport  Port=1
  mx chg pwr : Outport  Port=2
  mx dchg pwr : Outport  Port=3
  tag scope: ess_maxV_limited=global
  wires:
  Mux2/1 -> Imax chg=(Voc-Vmax)/R/1
  Iout/1 -> Max Chg current not exceeded/1, limit current based on  max voltage during charge/1, Max Dchg current not exceeded/1
  Imax chg=(Voc-Vmax)/R/1 -> Max Chg current not exceeded/2, Mux/1, limit current based on  max voltage during charge/3, Product/1
  Rchg/1 -> Mux2/2, Mux/2
  Voc/1 -> Mux2/1, Mux/3, Mux3/3, ess_module_num1/1
  Mux/1 -> Voc-I*R/1
  Voc-I*R/1 -> Product/2
  Product/1 -> mx chg pwr/1
  Max Chg current not exceeded/1 -> limit current based on  max voltage during charge/2, Logical Operator/1
  Logical Operator/1 -> [ess_maxV_limited]
  ess max voltage*#batts/1 -> Mux2/3
  limit current based on  max voltage during charge/1 -> limit current based on  min voltage during dcharge/3  "I_chgmax"
  limit current based on  min voltage during dcharge/1 -> Saturation/1, Limits/1(current req)
  Mux3/1 -> Imax dchg=(Voc -Vmin)/R/1, Vmin/1
  Imax dchg=(Voc -Vmin)/R/1 -> Saturation1/1
  ess max voltage*#batts1/1 -> limit by 0.5 battery  or min mc voltage  or ess min/3, Limits/6(V ess_min_volts)
  Rdchg/1 -> Mux3/1
  Max Dchg current not exceeded/1 -> limit current based on  min voltage during dcharge/2, Limits/2(current bat limited)
  mc min voltage/1 -> limit by 0.5 battery  or min mc voltage  or ess min/2, Limits/4(V mc_min_volts)
  ess_module_num1/1 -> limit by 0.5 battery  or min mc voltage  or ess min/1, Limits/5(V battery (.5Voc))
  limit by 0.5 battery  or min mc voltage  or ess min/1 -> Limits/3(V used), Mux3/2
  Vmin/1 -> Product1/2
  Product1/1 -> mx dchg pwr/1
  Saturation/1 -> Iout_lim/1
  Saturation1/1 -> Max Dchg current not exceeded/2, Product1/1, limit current based on  min voltage during dcharge/1

== system lib_energy_storage/Ess Choices/Ultracapacitor  System/ess tmp/Block NOTES ==
  note: This block models the thermal behavior of a battery module with active air cooling.
      | The module is modeled as a single lumped thermal mass.
      | The fan is on whenever the battery temp is > the set temp.

== system lib_energy_storage/Ess Choices/Ultracapacitor  System/ess tmp/Tair,ave ==
  Qess_case : Inport  Port=1  LatchInput=off
  Enable : EnablePort  StatesWhenEnabling=reset
  Block NOTES : Subsystem
      settings: RTWFcnNameOpts=Auto  RTWFileNameOpts=Auto
      mask Display: disp('Block\nNOTES')
  Tamb-(Q/mcp)/2 : Fcn  Expr=amb_tmp - (u(1)/(ess_mod_airflow*air_cp))/2
  do ex calcs?1 : Constant  Value=ess_th_res_on
  Tair_ave : Outport  Port=1  OutputWhenDisabled=reset  InitialOutput=amb_tmp
  Th Res : Outport  Port=2  OutputWhenDisabled=reset  InitialOutput=ess_th_res_off
  wires:
  Tamb-(Q/mcp)/2/1 -> Tair_ave/1
  Qess_case/1 -> Tamb-(Q/mcp)/2/1
  do ex calcs?1/1 -> Th Res/1

== system lib_energy_storage/Ess Choices/energy storage <ess>/ess tmp/Block NOTES ==
  note: This block models the thermal behavior of a battery module with active air cooling.
      | The module is modeled as a single lumped thermal mass.
      | The fan is on whenever the battery temp is > the set temp.

== system lib_energy_storage/Ess Choices/energy storage <ess>/ess tmp/Tair,ave ==
  Qess_case : Inport  Port=1  LatchInput=off
  Enable : EnablePort  StatesWhenEnabling=reset
  Block NOTES : Subsystem
      settings: RTWFcnNameOpts=Auto  RTWFileNameOpts=Auto
      mask Display: disp('Block\nNOTES')
  Tamb-(Q/mcp)/2 : Fcn  Expr=amb_tmp - (u(1)/(ess_mod_airflow*air_cp))/2
  do ex calcs?1 : Constant  Value=ess_th_res_on
  Tair_ave : Outport  Port=1  OutputWhenDisabled=reset  InitialOutput=amb_tmp
  Th Res : Outport  Port=2  OutputWhenDisabled=reset  InitialOutput=ess_th_res_off
  wires:
  do ex calcs?1/1 -> Th Res/1
  Qess_case/1 -> Tamb-(Q/mcp)/2/1
  Tamb-(Q/mcp)/2/1 -> Tair_ave/1

== system lib_energy_storage/Ess Choices/energy storage <ess>/limit power/Limits ==
  SOC  high limited : Inport  Port=1  LatchInput=off
  not SOC  low limited : Inport  Port=2  LatchInput=off
  power req : Inport  Port=3  LatchInput=off
  power bat limited : Inport  Port=4  LatchInput=off
  V used : Inport  Port=5  LatchInput=off
  V mc_min_volts : Inport  Port=6  LatchInput=off
  V battery (.5Voc) : Inport  Port=7  LatchInput=off
  V ess_min_volts : Inport  Port=8  LatchInput=off
  Logical Operator1 : Logic  Operator=NOT  Inputs=1
  Relational Operator{1,3..5} (4 alike) : RelationalOperator  Operator===
  limited by battery : Logic  Operator=AND  Inputs=2
  limited by battery min V : Logic  Operator=AND  Inputs=2
  limited by motor controller : Logic  Operator=AND  Inputs=2
  tag scope: ess_minV_limited=global, ess_pwr_limited=global, ess_soc_hi_limited=global, ess_soc_low_limited=global, mc_voltage_limited=global
  wires:
  SOC  high limited/1 -> [ess_soc_hi_limited]
  not SOC  low limited/1 -> Logical Operator1/1
  Logical Operator1/1 -> [ess_soc_low_limited]
  power req/1 -> Relational Operator1/1
  Relational Operator5/1 -> limited by battery min V/2
  Relational Operator4/1 -> limited by battery/2
  Relational Operator1/1 -> limited by battery min V/1, limited by battery/1, limited by motor controller/1
  Relational Operator3/1 -> limited by motor controller/2
  limited by battery min V/1 -> [ess_minV_limited]
  limited by battery/1 -> [ess_pwr_limited]
  limited by motor controller/1 -> [mc_voltage_limited]
  V ess_min_volts/1 -> Relational Operator5/2
  V battery (.5Voc)/1 -> Relational Operator4/2
  V used/1 -> Relational Operator5/1, Relational Operator4/1, Relational Operator3/1
  V mc_min_volts/1 -> Relational Operator3/2
  power bat limited/1 -> Relational Operator1/2

== system lib_energy_storage/Ess Choices/energy storage <ess>/max pack pwr (W)1/Rchg (ohms)1 ==
  x0 : Inport  Port=1  LatchInput=off
  y0 : Inport  Port=2  LatchInput=off
  Mux : Mux  Inputs=2
      settings: DisplayOption=none
  S-function : S-Function  FunctionName=sftable2  Parameters=xindex, yindex, table  PortCounts=[]  SFunctionModules=''
  table out : Outport  Port=1  InitialOutput=0
  wires:
  y0/1 -> Mux/2
  S-function/1 -> table out/1
  x0/1 -> Mux/1
  Mux/1 -> S-function/1

== system lib_energy_storage/Ess Choices/energy storage <ess>/max pack pwr (W)1/Rdis (ohms) ==
  x0 : Inport  Port=1  LatchInput=off
  y0 : Inport  Port=2  LatchInput=off
  Mux : Mux  Inputs=2
      settings: DisplayOption=none
  S-function : S-Function  FunctionName=sftable2  Parameters=xindex, yindex, table  PortCounts=[]  SFunctionModules=''
  table out : Outport  Port=1  InitialOutput=0
  wires:
  y0/1 -> Mux/2
  S-function/1 -> table out/1
  x0/1 -> Mux/1
  Mux/1 -> S-function/1

== system lib_energy_storage/Ess Choices/energy storage <ess>/max pack pwr (W)1/VOC (V) ==
  x0 : Inport  Port=1  LatchInput=off
  y0 : Inport  Port=2  LatchInput=off
  Mux : Mux  Inputs=2
      settings: DisplayOption=none
  S-function : S-Function  FunctionName=sftable2  Parameters=xindex, yindex, table  PortCounts=[]  SFunctionModules=''
  table out : Outport  Port=1  InitialOutput=0
  wires:
  y0/1 -> Mux/2
  S-function/1 -> table out/1
  x0/1 -> Mux/1
  Mux/1 -> S-function/1

== system lib_energy_storage/Ess Choices/energy storage <ess>/pack Voc, Rint/Rchg (ohms) ==
  x0 : Inport  Port=1  LatchInput=off
  y0 : Inport  Port=2  LatchInput=off
  Mux : Mux  Inputs=2
      settings: DisplayOption=none
  S-function : S-Function  FunctionName=sftable2  Parameters=xindex, yindex, table  PortCounts=[]  SFunctionModules=''
  table out : Outport  Port=1  InitialOutput=0
  wires:
  Mux/1 -> S-function/1
  x0/1 -> Mux/1
  S-function/1 -> table out/1
  y0/1 -> Mux/2
